simulink model "final_steady_24a"  (R2025a)
settings: Solver=ode15s  StartTime=0.0  StopTime=800  RelTol=1e-3
values from neighbouring files (symbols this model uses):
  A_rad = 100    [radiator_table.mat]
  bp_er = [1.0811 1.206647 1.332194 1.457741 1.583288 1.708835 1.834382 1.959929 2.085476 2.211022 2.336569 2.462116 ... (50 elements, 50x1)]    [turbine_table1.mat]
  bp_mf = [4.143 4.314878 4.486755 4.658633 4.83051 5.002388 5.174265 5.346143 5.51802 5.689898 5.861776 6.033653 ... (50 elements, 50x1)]    [turbine_table2.mat]
  bp_speed = [27545.65 33054.52 38563.39 44072.26 49581.13 55090 60598.87 66107.74]    [turbine_table1.mat]    (also in turbine_table2.mat)
  Cp_rad = 900    [radiator_table.mat]
  epsilon = 0.9    [radiator_table.mat]
  ETAT_table = [0.84155039588 0.848697265296 0.848208523418 0.846935956951 0.845688100512 0.844464241313 0.843263693717 0.842085797963 0.840929918951 0.839795445107 0.838681787297 0.83758837781 ... (624 elements, 12x52)]    [hexe_compressor_lookup.mat]
  h_h = 3000    [radiator_table.mat]
  M_rad = 500    [radiator_table.mat]
  m_ratio_bp = [0.870997765906 0.872298004303 0.875135300543 0.880934618207 0.883800006489 0.889571232111 0.892464712435 0.898207846014 0.901129418381 0.906844459918 0.909794124327 0.915481073822 ... (52 elements, 1x52)]    [hexe_compressor_lookup.mat]
  PR_table = [2.04199676148 2.45956167582 2.50151544166 2.54334896036 2.58604931564 2.62963124394 2.67410970466 2.71949988196 2.76581718659 2.81307725781 2.86129596521 2.91048941063 ... (624 elements, 12x52)]    [hexe_compressor_lookup.mat]
  speed_bp = [0.9 1 1.01 1.02 1.03 1.04 1.05 1.06 1.07 1.08 1.09 1.1]    [hexe_compressor_lookup.mat]
  table_eff = [0.8351 0.846857 0.858614 0.870372 0.882129 0.893886 0.903582 0.906405 0.909228 0.912051 0.914875 0.917698 ... (400 elements, 50x8)]    [turbine_table2.mat]
  table_mf = [4.143 7.751628 9.52994 10.565952 11.261817 11.739474 12.104735 12.304118 12.503501 12.565 12.565 12.565 ... (400 elements, 50x8)]    [turbine_table1.mat]
  theta = 5.67e-08    [radiator_table.mat]
(part 2 of 2)

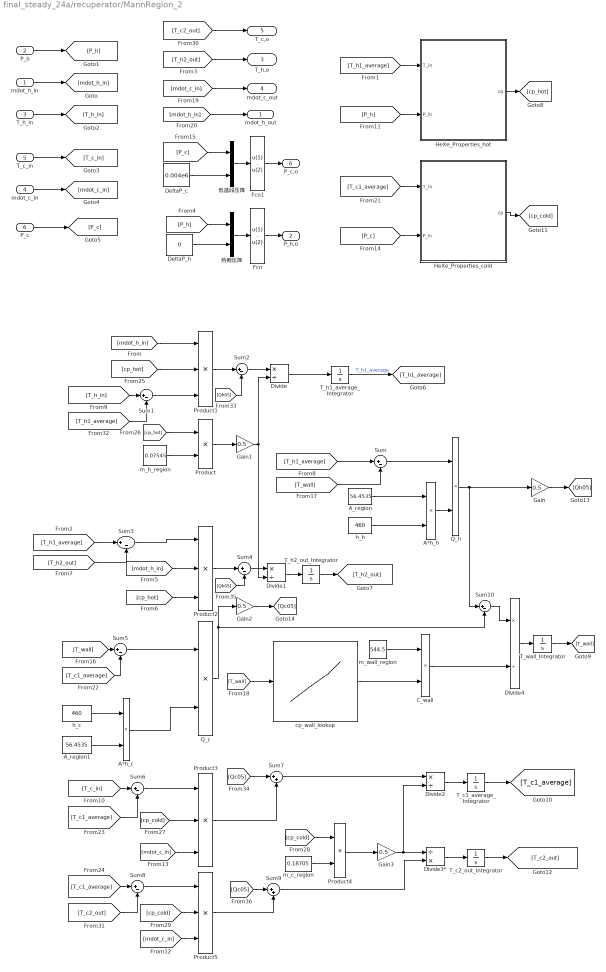
== system final_steady_24a/recuperator/MannRegion_2 ==
  mdot_h_in : Inport
  P_h : Inport  Port=2
  T_h_in : Inport  Port=3
  mdot_c_in : Inport  Port=4
  T_c_in : Inport  Port=5
  P_c : Inport  Port=6
  A*h_c : Product
  A*h_h : Product
  A_region : Constant  Value=56.4535
  A_region1 : Constant  Value=56.4535
  C_wall : Product
  DeltaP_c : Constant  Value=0.004e6
  DeltaP_h : Constant  Value=0
  Divide{,1..2,4} (4 alike) : Product  Inputs=*/
  Divide3* : Product  Inputs=/*
  Fcn : Fcn  Expr=u(1) - u(2)
  Fcn1 : Fcn  Expr=u(1) - u(2)
  Gain{,1..3} (4 alike) : Gain  Gain=0.5
  HeXe_Properties_cold : MATLAB Function  TreatAsAtomicUnit=on
  HeXe_Properties_hot : MATLAB Function  TreatAsAtomicUnit=on
  Product : Product
  Product{1..3,5} (4 alike) : Product  Inputs=3
  Product4 : Product
  Q_c : Product
  Q_h : Product
  Sum{,1..6,8,10} (9 alike) : Sum  Inputs=|+-
  Sum7 : Sum  Inputs=|++
  Sum9 : Sum  Inputs=|++
  T_c1_average_Integrator : Integrator  InitialCondition=702.613837679092
  T_c2_out_Integrator : Integrator  InitialCondition=814.166559982758
  T_h1_average_Integrator : Integrator  InitialCondition=809.582867595475
  T_h2_out_Integrator : Integrator  InitialCondition=697.991790217874
  T_wall_Integrator : Integrator  InitialCondition=756.098352685598
  cp_wall_lookup : Lookup_n-D  NumberOfTableDimensions=1  BreakpointsForDimension1=[293.15, 373.15, 473.15, 573.15, 673.15,773.15, 873.15, 973.15, 1073.15, 1173.15,1273.15]  Table=[419, 440, 465, 490, 515,536, 561, 586, 611, 636, 662]  InternalRulePriority=Speed  RndMeth=Simplest
  h_c : Constant  Value=460
  h_h : Constant  Value=460
  m_c_region : Constant  Value=0.18705
  m_h_region : Constant  Value=0.07545
  m_wall_region : Constant  Value=544.5
  低温段压降 : Mux  Inputs=2
  热侧压降 : Mux  Inputs=2
  mdot_h_out : Outport
  P_h,o : Outport  Port=2
  T_h,o : Outport  Port=3
  mdot_c_out : Outport  Port=4
  T_c,o : Outport  Port=5
  P_c,o : Outport  Port=6
  wires:
  mdot_c_in/1 -> [mdot_c_in]
  mdot_h_in/1 -> [mdot_h_in]
  T_h1_average_Integrator/1 -> [T_h1_average]  "T_h1_average"
  T_wall_Integrator/1 -> [T_wall]
  A_region/1 -> A*h_h/1
  h_h/1 -> A*h_h/2
  A*h_h/1 -> Q_h/2
  T_h_in/1 -> [T_h_in]
  Sum1/1 -> Product1/3
  Q_h/1 -> Gain/1, Sum10/1
  Product1/1 -> Sum2/1
  Gain/1 -> [Qh05]
  m_h_region/1 -> Product/2
  Product/1 -> Gain1/1
  Sum2/1 -> Divide/1
  Gain1/1 -> Divide/2, Divide1/2
  Divide/1 -> T_h1_average_Integrator/1
  T_h2_out_Integrator/1 -> [T_h2_out]
  Sum3/1 -> Product2/1
  Product2/1 -> Sum4/1
  Sum4/1 -> Divide1/1
  Divide1/1 -> T_h2_out_Integrator/1
  T_c1_average_Integrator/1 -> [T_c1_average]
  h_c/1 -> A*h_c/1
  A*h_c/1 -> Q_c/2
  Sum5/1 -> Q_c/1
  T_c_in/1 -> [T_c_in]
  Q_c/1 -> Gain2/1, Sum10/2
  Gain2/1 -> [Qc05]
  Product3/1 -> Sum7/2
  m_c_region/1 -> Product4/2
  Sum7/1 -> Divide2/1
  Gain3/1 -> Divide2/2, Divide3*/1
  Divide2/1 -> T_c1_average_Integrator/1
  T_c2_out_Integrator/1 -> [T_c2_out]
  Sum8/1 -> Product5/1
  Product5/1 -> Sum9/2
  Sum9/1 -> Divide3*/2
  Divide3*/1 -> T_c2_out_Integrator/1
  m_wall_region/1 -> C_wall/1
  C_wall/1 -> Divide4/2
  Sum10/1 -> Divide4/1
  Divide4/1 -> T_wall_Integrator/1
  Sum6/1 -> Product3/1
  P_h/1 -> [P_h]
  P_c/1 -> [P_c]
  cp_wall_lookup/1 -> C_wall/2
  DeltaP_c/1 -> 低温段压降/2
  DeltaP_h/1 -> 热侧压降/2
  Fcn/1 -> P_h,o/1
  热侧压降/1 -> Fcn/1
  低温段压降/1 -> Fcn1/1
  Fcn1/1 -> P_c,o/1
  [mdot_h_in] -> Product1/1
  [T_h1_average] -> Sum3/1
  [T_h2_out] -> T_h,o/1
  [P_h] -> 热侧压降/1
  [mdot_h_in] -> Product2/2
  [cp_hot] -> Product2/3
  [T_h2_out] -> Sum3/2
  [T_h1_average] -> Sum/1
  [T_h_in] -> Sum1/1
  [T_c_in] -> Sum6/1
  [mdot_c_in] -> Product5/3
  [mdot_c_in] -> Product3/3
  [P_c] -> 低温段压降/1
  [T_wall] -> Sum5/1
  [T_wall] -> Sum/2
  [T_wall] -> cp_wall_lookup/1
  A_region1/1 -> A*h_c/2
  Sum/1 -> Q_h/1
  [mdot_c_in] -> mdot_c_out/1
  [mdot_h_in] -> mdot_h_out/1
  [T_c1_average] -> Sum5/2
  [T_c1_average] -> Sum6/2
  [T_c1_average] -> Sum8/1
  [cp_hot] -> Product1/2
  [cp_hot] -> Product/1
  [cp_cold] -> Product3/2
  [cp_cold] -> Product4/1
  [cp_cold] -> Product5/2
  [T_c2_out] -> T_c,o/1
  [T_c2_out] -> Sum8/2
  [T_h1_average] -> Sum1/2
  Product4/1 -> Gain3/1
  [Qh05] -> Sum2/2
  [Qh05] -> Sum4/2
  [Qc05] -> Sum7/1
  [Qc05] -> Sum9/1
  HeXe_Properties_cold/1(cp) -> [cp_cold]
  [P_h] -> HeXe_Properties_hot/2(P_in)
  [T_c1_average] -> HeXe_Properties_cold/1(T_in)
  [P_c] -> HeXe_Properties_cold/2(P_in)
  [T_h1_average] -> HeXe_Properties_hot/1(T_in)
  HeXe_Properties_hot/1(cp) -> [cp_hot]

== system final_steady_24a/rediator/Subsystem ==
  Constant : Constant  Value=epsilon
  Constant1 : Constant  Value=theta
  Constant2 : Constant  Value=A_rad
  Constant3 : Constant  Value=M_rad
  Constant4 : Constant  Value=Cp_rad
  Constant5 : Constant  Value=h_h
  epsilon : Outport
  theta : Outport  Port=2
  A_rad : Outport  Port=3
  M_rad : Outport  Port=4
  Cp_rad : Outport  Port=5
  h_h : Outport  Port=6
  wires:
  Constant3/1 -> M_rad/1
  Constant5/1 -> h_h/1
  Constant2/1 -> A_rad/1
  Constant1/1 -> theta/1
  Constant/1 -> epsilon/1
  Constant4/1 -> Cp_rad/1

== system final_steady_24a/TAC/Turbine/Pressure Drop ==
  2-3 : Constant  Value=0
  3-4 : Constant  Value=0.011605
  5-6 : Constant  Value=0.005158
  6-1 : Constant  Value=0.002579
  constant : Constant
  1 : Outport
  p5-6 : Outport  Port=2
  p6-1 : Outport  Port=3
  p2-3 : Outport  Port=4
  p3-4 : Outport  Port=5
  wires:
  5-6/1 -> p5-6/1
  3-4/1 -> p3-4/1
  constant/1 -> 1/1
  6-1/1 -> p6-1/1
  2-3/1 -> p2-3/1

== matlab function final_steady_24a/IHX/IHX_region_1/HeXe_Properties_cold ==
  data: T_c1_average input; cp output; P_in input
function cp = HeXe_Properties_cold(T_c1_average,P_in)

coder.extrinsic('HeXe_property_simulink');

cp = 0;
[cp, ~, ~, ~, ~, ~] = ...
    HeXe_property_simulink(T_c1_average, P_in);
end

== matlab function final_steady_24a/IHX/IHX_region_1/Lithium_Properties_hot ==
  data: T_h1_average input; P_c input; cp output
function cp = Lithium_Properties_hot(T_h1_average, P_c)
% 热侧液锂比热容。
% 为保持原有两个输入端口和连线不变，保留 P_c；
% 液锂物性使用设计压力 0.234 MPa。

coder.extrinsic('Lithium_property_simulink');

cp = 0;
[cp, ~, ~, ~, ~, ~] = ...
    Lithium_property_simulink(T_h1_average, 0.234e6);
end

== matlab function final_steady_24a/IHX/IHX_region_2/Lithium_Properties_hot ==
  data: T_h1_average input; P_c input; cp output
function cp = Lithium_Properties_hot(T_h1_average, P_c)
% 热侧液锂比热容。
% 为保持原有两个输入端口和连线不变，保留 P_c；
% 液锂物性使用设计压力 0.234 MPa。

coder.extrinsic('Lithium_property_simulink');

cp = 0;
[cp, ~, ~, ~, ~, ~] = ...
    Lithium_property_simulink(T_h1_average, 0.234e6);
end

== matlab function final_steady_24a/TAC/Compressor/HeXe_Properties (point 1) ==
  data: T_in input; P_in input; gamma output
function gamma = HeXe_Properties_hot(T_in, P_in)
coder.extrinsic('HeXe_property_simulink');
gamma=0;
[~, gamma, ~, ~, ~, ~] = HeXe_property_simulink(T_in, P_in);
end

== matlab function final_steady_24a/IHX/IHX_region_2/HeXe_Properties_cold ==
  data: T_c1_average input; cp output; P_in input
function cp = HeXe_Properties_cold(T_c1_average,P_in)

coder.extrinsic('HeXe_property_simulink');

cp = 0;
[cp, ~, ~, ~, ~, ~] = ...
    HeXe_property_simulink(T_c1_average, P_in);
end

== matlab function final_steady_24a/TAC/Compressor/HeXe_Properties(point 1)1 ==
  data: T_in input; P_in input; cp1 output
function cp1 = HeXe_Properties(T_in, P_in)
coder.extrinsic('HeXe_property_simulink');
cp1 = 0; 
[cp1, ~, ~, ~, ~, ~] = HeXe_property_simulink(T_in, P_in);
end

== matlab function final_steady_24a/TAC/Compressor/HeXe_Properties(point 2s) ==
  data: T5s input; P_out input; cp2 output
function cp2 = HeXe_Properties(T5s, P_out)
coder.extrinsic('HeXe_property_simulink');
cp2 = 0; 
[cp2, ~, ~, ~, ~, ~] = HeXe_property_simulink(T5s, P_out);
end

== matlab function final_steady_24a/TAC/Compressor/MATLAB Function ==
  data: T_in input; r input; T5s output; gamma input
function T5s = fcn(T_in, r, gamma)
T5s = T_in * r^((gamma - 1)/gamma);
end

== matlab function final_steady_24a/recuperator/MannRegion_1/HeXe_Properties_cold ==
  data: T_in input; P_in input; cp output
function cp = HeXe_Properties_cold(T_in, P_in)
% 调用外置函数计算 He-Xe 比热容
coder.extrinsic('HeXe_property_simulink');

cp = 0;                                     % 必须先初始化
[cp, ~, ~, ~, ~, ~] = HeXe_property_simulink(T_in, P_in);  % 调用外部文件
end

== matlab function final_steady_24a/recuperator/MannRegion_1/HeXe_Properties_hot ==
  data: T_in input; P_in input; cp output
function cp = HeXe_Properties_hot(T_in, P_in)
% 调用外置函数计算 He-Xe 比热容
coder.extrinsic('HeXe_property_simulink');

cp = 0;                                     % 必须先初始化
[cp, ~, ~, ~, ~, ~] = HeXe_property_simulink(T_in, P_in);  % 调用外部文件
end

== matlab function final_steady_24a/recuperator/MannRegion_2/HeXe_Properties_cold ==
  data: T_in input; P_in input; cp output
function cp = HeXe_Properties_cold(T_in, P_in)
% 调用外置函数计算 He-Xe 比热容
coder.extrinsic('HeXe_property_simulink');

cp = 0;                                     % 必须先初始化
[cp, ~, ~, ~, ~, ~] = HeXe_property_simulink(T_in, P_in);  % 调用外部文件
end

== matlab function final_steady_24a/recuperator/MannRegion_2/HeXe_Properties_hot ==
  data: T_in input; P_in input; cp output
function cp = HeXe_Properties_hot(T_in, P_in)
% 调用外置函数计算 He-Xe 比热容
coder.extrinsic('HeXe_property_simulink');

cp = 0;                                     % 必须先初始化
[cp, ~, ~, ~, ~, ~] = HeXe_property_simulink(T_in, P_in);  % 调用外部文件
end

== matlab function final_steady_24a/TAC/Compressor/MATLAB Function1 ==
  data: T_out output; T_in input; eta_c input; cp1 input; cp2 input; T5s input
function T_out = Fcn(T_in, eta_c, cp1, cp2, T5s)
T_out = T_in + (cp2*(T5s - T_in))/(cp1*eta_c);
end

== matlab function final_steady_24a/precooler/precooler_1/HeXe_Properties_hot ==
  data: T_in input; P_in input; cp output
function cp = HeXe_Properties_hot(T_in, P_in)
% 调用外置函数计算 He-Xe 比热容
coder.extrinsic('HeXe_property_simulink');

cp = 0;                                     % 必须先初始化
[cp, ~, ~, ~, ~, ~] = HeXe_property_simulink(T_in, P_in);  % 调用外部文件
end

== matlab function final_steady_24a/precooler/precooler_1/NaK_Properties_cold ==
  data: T_in input; cp output
function cp = NaK_Properties_cold(T_in)
cp = 1000.*(1.061 - 3.694e-4.*T_in + 4.615e-8.*T_in.^2 + 1.509e-10.*T_in.^3);
end

== matlab function final_steady_24a/precooler/precooler_2/HeXe_Properties_hot ==
  data: T_in input; P_in input; cp output
function cp = HeXe_Properties_hot(T_in, P_in)
% 调用外置函数计算 He-Xe 比热容
coder.extrinsic('HeXe_property_simulink');

cp = 0;                                     % 必须先初始化
[cp, ~, ~, ~, ~, ~] = HeXe_property_simulink(T_in, P_in);  % 调用外部文件
end

== matlab function final_steady_24a/precooler/precooler_2/NaK_Properties_cold1 ==
  data: T_in input; cp output
function cp = NaK_Properties_cold(T_in)
cp = 1000.*(1.061 - 3.694e-4.*T_in + 4.615e-8.*T_in.^2 + 1.509e-10.*T_in.^3);
end

== matlab function final_steady_24a/rediator/MATLAB Function ==
  data: T input; Cp output
function Cp = Cp_h(T)
Cp = 1000.*(1.061 - 3.694e-4.*T + 4.615e-8.*T.^2 + 1.509e-10.*T.^3);
end

== matlab function final_steady_24a/TAC/Turbine/HeXe_Properties (point 1) ==
  data: T_in input; P_in input; gamma output
function gamma = HeXe_Properties_hot(T_in, P_in)
% 调用外置函数计算 He-Xe 比热容
coder.extrinsic('HeXe_property_simulink');
gamma=0;
[~, gamma, ~, ~, ~, ~] = HeXe_property_simulink(T_in, P_in);  % 调用外部文件
end

== matlab function final_steady_24a/TAC/Turbine/HeXe_Properties(point 1) ==
  data: T_in input; P_in input; cp1 output
function cp1 = HeXe_Properties(T_in, P_in)
% 调用外置函数计算 He-Xe 比热容
coder.extrinsic('HeXe_property_simulink');
cp1 = 0; 
[cp1, ~, ~, ~, ~, ~] = HeXe_property_simulink(T_in, P_in);  % 调用外部文件
end

== matlab function final_steady_24a/TAC/Turbine/HeXe_Properties(point 2s) ==
  data: T_in input; P_in input; cp2 output
function cp2 = HeXe_Properties(T_in, P_in)
% 调用外置函数计算 He-Xe 比热容
coder.extrinsic('HeXe_property_simulink');
cp2 = 0; 
[cp2, ~, ~, ~, ~, ~] = HeXe_property_simulink(T_in, P_in);  % 调用外部文件
end

== matlab function final_steady_24a/TAC/Turbine/MATLAB Function ==
  data: pi input; T2s output; phi input; T1 input
function T2s = fcn(pi, phi, T1)
    T2s = T1 * pi^(-phi);
end

== matlab function final_steady_24a/TAC/Turbine/MATLAB Function1 ==
  data: T2 output; T1 input; neta input; cp1 input; cp2 input; T2s input
function T2= Fcn(T1,neta,cp1,cp2,T2s)
T2=T1-(neta*cp2*(T1-T2s))/cp1;
end
